simulink model "LFC_model"  (R2020b)
settings: Solver=VariableStepAuto  StartTime=0.0  StopTime=20  FixedStep=0.001  MaxStep=0.01  RelTol=1e-3
values from neighbouring files (symbols this model uses):
  Kg = 1    [LFC_parameters.m]
  Ki = (1/(4*Kp*Tp)) * (1+(Kp/R))^2    (= 0.325125)    [LFC_parameters.m]
  Kp = 1/D    (= 100)    [LFC_parameters.m]
  Kt = 1    [LFC_parameters.m]
  R = R * nominal_freq    (= 2)    [LFC_parameters.m]
  Tg = 0.08    [LFC_parameters.m]
  Tp = (2*H) / (nominal_freq * D)    (= 20)    [LFC_parameters.m]
  Tt = 0.3    [LFC_parameters.m]
libraries: simulink x4
settings Model: Creator=mapez  LastModifiedBy=mapez

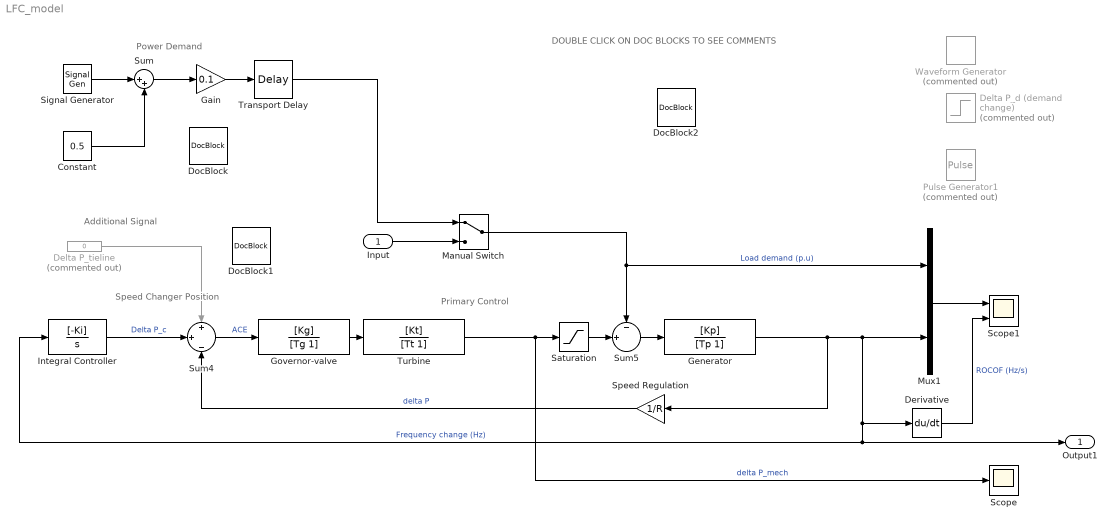
== system LFC_model ==
  note: DOUBLE CLICK ON DOC BLOCKS TO SEE COMMENTS
  note: Speed
      | Changer
      | Position
  note: Power Demand
  note: Primary Control
  note: Additional Signal
  Input : Inport
  Constant : Constant  Value=0.5
  Delta P_d (demand change) : Step  Commented=on  After=0.162  SampleTime=0
  Delta P_tieline : Constant  Commented=on  Value=0
  Derivative : Derivative
  DocBlock : simulink/Model-Wide Utilities/DocBlock  DocumentType=Text
      content=|
      | This is symply a signal generator to model the load demand.
      | The transport delay block is simply for plotting convenience,
      | and the gain block sets the amplitude per-unit.
      |
      | You can open the signal generator block to change the waveform
      | and frequency. The resonant frequency is around 2.27 rads/s as
      | seen in the bode plot.
  DocBlock1 : simulink/Model-Wide Utilities/DocBlock  DocumentType=Text
      content=|
      | Not used in this model, this is to introduce tie-line power in
      | multi-area simulations.
  DocBlock2 : simulink/Model-Wide Utilities/DocBlock  DocumentType=Text
      content=|
      | This model simulates a generic single area LFC system with
      | primary and secondary integral control.
      |
      | System parameters are from a typical system and sourced from:
      | https://www.researchgate.net/publication/222227238_AGC_for_autonomous_power_system_using_combined_intelligent_techniques
      |
      | You must run the script LFC_parameters.m beforehand to have the
      | relevant system parameters in the workspace.
      |
      | To run the model manually make sure the manual switch connects
      | the power demand area (blue) and examine scopes.
      |
      | To linearize the model make sure the manual switch connects the
      | input block (red). To linearize either:
      |
      | * Open the Model Linearizer App and select "Root level Inports
      | and Outports" under "Analysis I/Os".
      |
      | * Or run the LFC_linearized.m script.
      |
      | The latter automatically displays step and impulse responses,
      | pole-zero map, Bode, Nyquist, and Nichols plots.
  Gain : Gain  Gain=0.1
  "Generator " : TransferFcn  Numerator=[Kp]  Denominator=[Tp 1]
  "Governor-valve " : TransferFcn  Numerator=[Kg]  Denominator=[Tg 1]
  Integral Controller : TransferFcn  Numerator=[-Ki]  Denominator=[1 0]
  Manual Switch : ManualSwitch
  Mux1 : Mux  Inputs=2
  Pulse Generator1 : DiscretePulseGenerator  Commented=on  PulseType=Time based  Amplitude=0.1  Period=2*pi/2.27  PulseWidth=50  PhaseDelay=1
  Saturation : Saturate
  Scope : Scope
  Scope1 : Scope  NumInputPorts=2
  Signal Generator : SignalGenerator  WaveForm=square  Amplitude=0.5  Frequency=2.27  Units=rad/sec
  Speed Regulation : Gain  Gain=1/R
  Sum : Sum  Inputs=|++
  Sum4 : Sum  Inputs=+|+|-
  Sum5 : Sum  Inputs=-|+||
  Transport Delay : TransportDelay
  "Turbine " : TransferFcn  Numerator=[Kt]  Denominator=[Tt 1]
  Waveform Generator : simulink/Sources/Waveform Generator  Commented=on  OutMin=[]  OutMax=[]  OutDataTypeStr=double  SelectedSignal=1  Signals=sin(0.01, 50, 90)  BlockNames=MultiportSwitch_94a09d222338447  SampleTime=0.1
  Output1 : Outport
  wires:
  Delta P_tieline/1 -> Sum4/1
  Speed Regulation/1 -> Sum4/3  "delta P"
  "Turbine "/1 -> Saturation/1, Scope/1  "delta P_mech"
  Sum4/1 -> "Governor-valve "/1  "ACE"
  Mux1/1 -> Scope1/1
  Sum5/1 -> "Generator "/1
  "Governor-valve "/1 -> "Turbine "/1
  "Generator "/1 -> Speed Regulation/1, Mux1/2, Output1/1, Integral Controller/1, Derivative/1  "Frequency change (Hz)"
  Integral Controller/1 -> Sum4/2  "Delta P_c"
  Derivative/1 -> Scope1/2  "ROCOF (Hz/s)"
  Signal Generator/1 -> Sum/1
  Constant/1 -> Sum/2
  Sum/1 -> Gain/1
  Manual Switch/1 -> Sum5/1, Mux1/1  "Load demand (p.u)"
  Input/1 -> Manual Switch/2
  Gain/1 -> Transport Delay/1
  Saturation/1 -> Sum5/2
  Transport Delay/1 -> Manual Switch/1
